simulink model "wamjc7"  (Simulink 8.3)
settings: Solver=ode4  SolverMode=SingleTasking  StartTime=0.0  StopTime=inf  FixedStep=sample_time  RelTol=1e-3
undefined symbols (not defined in the file): arm_home, arm_home_norest, arm_j2mt, arm_m2jp, b, bit, C, CAN_init, enc_per_rev, FT_init, hand_on, MT_init, puck_I_per_Nm, rotFT2Hand, sample_time, Standard, VL1_init, VL2_init
libraries: xpclib x43, simulink x27, xpcutilitieslib x6, dspmathops x1, dspadpt3 x1, dspindex x1, dspbuff3 x1
(part 4 of 5)

== matlab function Get Arm State/Get Gripper Status/Grasp Success ==
  data: isGraspMessage input double; grasp_success output double; errorcode input double
function grasp_success = f(isGraspMessage, errorcode)
%#eml

    persistent errorcode_last;
    
    if isempty(errorcode_last)
       errorcode_last = -1; 
    end

    grasp_success = 0;
    
    % If this is a grasp message, the current errorcode is a grasp succces 
    % and the previous one was not then return a success
    if isGraspMessage && errorcode == 0 && errorcode_last ~= 0
       grasp_success = 1; 
       errorcode_last = double(errorcode);
    elseif ~isGraspMessage
        errorcode_last = -1;
    end
    

end

== matlab function Subsystem/Plan Arm Trajectory/Determine parameters ==
  data: dt input double; x0 output double; xf output double; acc output double; vel output double; Tdes output double; pos output double; hand_on input double; x0_in input double; pckt input double; type output double; guarded output double; FT input double
% if joint space move, computes the trajectory using a trapezoidal velocity profile
% if cartesian space move, computes the trajectory using one selected position axis, and theta

% if joint space:
% x0,xf are start and end position in radians
%     type==0
% if cartesian space:
% x0,xf are start and end position in meters/radians
%     type==any other
function [x0,xf,acc,vel,Tdes,pos,type, guarded] = det_params(dt,hand_on,x0_in,pckt,FT)

    % This is used for compliant closing
    persistent initialGripperWidth;
    
    if(isempty(initialGripperWidth))
        initialGripperWidth = 0;
    end
    
    % parse the UDP packet
    % pckt(1) is a double but is converted to uint8 (mask1 mask2 mask3 mask4 mask5 type(3 bits))
    data = uint8(pckt(1));
    bits = bitand(bitshift(data,-7:0),1)';
    posMask = 2*bits(4)+bits(5);
    
    type = double(4*bits(6)+2*bits(7)+bits(8));
    guarded = [0 0 dt 0 0];
    % determine x0 (depends on cartesian space or joint space)
    % joint space move
    if(type == 0)
        acc = pckt(9:15);
        vel = pckt(16:22);
        xf  = pckt(2:8);
        
        Tdes = nan(4,4);
        x0 = x0_in;
        pos = nan(3,1);
        guarded = [0 0 dt 0 0];
    % cartesian space move
    elseif(type == 1)
        % acc and vel are unused for Jacobian Transpose controller
        acc = [.05 .05 .05 .05 0 0 0]';
        vel = [.1  .1  .1  .1  0 0 0]';
        % Unpack the transfomation matrix
        TF = [pckt(2)  pckt(3)  pckt(4)  pckt(5);
              pckt(6)  pckt(7)  pckt(8)  pckt(9);
              pckt(10) pckt(11) pckt(12) pckt(13);
              0 0 0 1;];
        Tdes = TF; % Entire transformation matrix describing desired tool configuration
        
        % Build the guarded signal from the packet
        guarded = [pckt(18) pckt(19) dt pckt(20) pckt(21)];
        
        pos = TF(1:3,4);  % Position part of transformation matrix describing the desired tool configuration
        
        % we need to compute the forward kinematics
        % to determine the initial tool configuration vector
        
        % a, d, and alpha (b) DH parameters
        dh_a = [0 0 0.045 -0.045 0 0 0 0];
        dh_d = [0 0 0.55 0 0.3 0 .061 0]; % Not sure about dh_d(8) For the hand
        dh_b = [-pi/2 pi/2 -pi/2 pi/2 -pi/2 pi/2 0 0];

        % hand on
        if (hand_on)
            dh_d(8) = 0.0953; % Schunk Gripper
        end

        % compute forward kinematics of initial position
        ct = cos([x0_in; 0]);
        st = sin([x0_in; 0]);
        cb = cos(dh_b);
        sb = sin(dh_b);        
        T0 = eye(4);
        for i=1:8
            T = [ ct(i), -st(i)*cb(i),  st(i)*sb(i), dh_a(i)*ct(i);
                  st(i),  ct(i)*cb(i), -ct(i)*sb(i), dh_a(i)*st(i);
                  0, sb(i), cb(i), dh_d(i);
                  0, 0, 0, 1 ];
            T0 = T0*T;
        end
        
        x0 = [T0(1:3,4)' 0 0 0 0]';
        xf = [pos' 0 0 0 0]';

    % A Trajectory Move
    elseif(type == 2)
        % Execute a trajectory given in the UDP packet.  There will be 100 points along the trajectory,
        % each with seven values (joints 1-7).  In the packet the points will start at pckt(PTS_START)
        
        acc = zeros(7,1);
        vel = zeros(7,1);
        pos = zeros(3,1);
        x0 = zeros(7,1);
        xf = zeros(7,1);
        
        PTS_START = 3;  

        % Get the length (in seconds) that the trajectory should take
        trajectoryEndTime = pckt(2);
        
        % Index of 100 points in the trajectory that the current time falls at
        index = (dt / trajectoryEndTime)*100;
        % The first point that we will want to interpolate between
        lowIndex = floor(index);
        % The distance between the two points (used for linear interpolation)
        alpha = index - lowIndex;
        
        % Get the start and end joint angles from the packet
        startIndex = lowIndex*7 + PTS_START;
        qStart = zeros(1,7);
        qEnd = zeros(1,7);
        qStart(1) = pckt(startIndex    );
        qStart(2) = pckt(startIndex + 1);
        qStart(3) = pckt(startIndex + 2);
        qStart(4) = pckt(startIndex + 3);
        qStart(5) = pckt(startIndex + 4);
        qStart(6) = pckt(startIndex + 5);
        qStart(7) = pckt(startIndex + 6);
        qEnd(1)   = pckt(startIndex + 7);
        qEnd(2)   = pckt(startIndex + 8);
        qEnd(3)   = pckt(startIndex + 9);
        qEnd(4)   = pckt(startIndex + 10);
        qEnd(5)   = pckt(startIndex + 11);
        qEnd(6)   = pckt(startIndex + 12);
        qEnd(7)   = pckt(startIndex + 13);

        % For some reason Matlab did not like the syntax:
        %  qStart = pckt(startIndex : startIndex + 6);
        %  qEnd   = pckt(startIndex + 7 : startIndex + 13);
        % or even
        %  qStart(1:7) = pckt(startIndex : startIndex + 6);
        
        % Do a linear interpolation between the two joint angles
        qdes = (1-alpha)*qStart + alpha*qEnd;
        
        %Pack the position into Tdes so we do not have to create another signal
        Tdes = zeros(4,4);
        Tdes(1:7) = qdes';
        
        % Put finised time in x0(1)
        x0(1) = trajectoryEndTime;
        
    % Compliant close.
    elseif type == 3       
        x0 = zeros(7,1);
        xf = zeros(7,1);
        acc = zeros(7,1);
        vel = zeros(7,1);
        pos = zeros(3,1);
        
        % If we are just at the beginning of a compliant close, get the
        % current gripper width as the starting gripper width
        if dt < .004
           %initialGripperWidth = FT(8); 
           initialGripperWidth = .1;
        end
        
        targetGripperWidth = pckt(2);
        gripperSpeed = pckt(3);
        finger = pckt(4);
        
        totalTime = abs(initialGripperWidth - targetGripperWidth) / gripperSpeed;
        
        % Get the fingertip position
        fingerTipPosition = finger*initialGripperWidth/2;
                
        % a, d, and alpha (b) DH parameters
        dh_a = [0 0 0.045 -0.045 0 0 0 0];
        dh_d = [0 0 0.55 0 0.3 0 .061 0]; % Not sure about dh_d(8) For the hand
        dh_b = [-pi/2 pi/2 -pi/2 pi/2 -pi/2 pi/2 0 0];

        % hand on
        if (hand_on)
            dh_d(8) = 0.0953; % Schunk Gripper
        end

        % compute forward kinematics of initial position
        ct = cos([x0_in; 0]);
        st = sin([x0_in; 0]);
        cb = cos(dh_b);
        sb = sin(dh_b);
        T0 = eye(4);
        for i=1:8
            T = [ ct(i), -st(i)*cb(i),  st(i)*sb(i), dh_a(i)*ct(i);
                  st(i),  ct(i)*cb(i), -ct(i)*sb(i), dh_a(i)*st(i);
                  0, sb(i), cb(i), dh_d(i);
                  0, 0, 0, 1 ];
            T0 = T0*T;
        end
        
        % Add the rotated vector from palm to fingertip
        T0(1:3,4) = T0(1:3,4) + T0(1:3,1:3)*[0;fingerTipPosition;.073];
        
        Tdes = T0;
        
        % Build the guarded signal
        guarded = [0 0 dt 0 0];
        
        % Get the time that the gripper should take to close
        x0(1) = totalTime;
        
        % The grasp success flag
        x0(2) = FT(9);
        
        % pos(1) pass which finger should remain stationary through to the
        % compute qdes,qddes block
        pos(1) = finger;
        
        % pos(2) holds the predicted gripper position
        pos(2) = initialGripperWidth - (dt/totalTime)*(initialGripperWidth - targetGripperWidth);
    elseif type == 5
        x0 = x0_in;
        xf = x0_in;
        acc = zeros(7,1);
        vel = zeros(7,1);
        Tdes = zeros(4,4);
        pos = zeros(3,1);
        guarded = [0 0 dt 0 0];
        vel(1) = pckt(2);  % Tf for an impedance move
    else
        x0 = x0_in;
        xf = x0_in;
        acc = zeros(7,1);
        vel = zeros(7,1);
        Tdes = zeros(4,4);
        pos = zeros(3,1);
        %type = 0;
    end
end

== matlab function Subsystem/Plan Arm Trajectory/Trapezoidal Profile2 ==
  data: dt input double; xdes output double; x0 input double; xf input double; acc input double; vel input double; xddes output double; done output double; type input double; cartesian_error input double; m output double
function [xdes,xddes,done,m] = trap_traj(dt,x0,xf,acc,vel,type,cartesian_error)
    % assume we're done
    done = 1;

    % initialize xdes and xddes
    xdes = zeros(7,1);
    xddes = zeros(7,1);
    m = [0.0 0.0 dt];

    if type == 0
        % iterate through joints
        for i=1:7
            % check if we're already done with this joint
            if(xf(i) == x0(i))
                xdes(i) = xf(i);
                % xddes(i) was initialized to 0
                continue;
            end

            % change acceleration and velocity to appropriate sign
            a = acc(i)*sign(xf(i)-x0(i));
            v = vel(i)*sign(xf(i)-x0(i));

            % t1,q1 are the time and position at the first peak of the trapezoid
            % t2,q2 are the time and position at the second peak of the trapezoid
            % v2 is the velocity at the midpoint of the trapezoid
            % qramp is the distance traveled during the acceleration phase
            % tmid is the time spent at constant velocity
            % tf is the total time to reach desired position (t1+t2+tmid)
            % a = vt; q = 0.5*a*t^2
            t1 = v/a;
            qramp = 0.5*a*t1^2;

            % acceleration is not high enough to reach our constant velocity, so trapezoid
            % looks like a triangle instead
            if (abs(2*qramp) > abs(xf(i)-x0(i)))
                % (xf-x0)/2 = 0.5*a*t^2
                t1 = sqrt((xf(i)-x0(i))/a);
                tmid = 0;
                qramp = (xf(i)-x0(i))/2;
                v2 = a*t1;
            % we will hit constant velocity, so trapezoid is really a trapezoid
            else
                tmid = (xf(i)-x0(i)-2*qramp)/v;
                v2 = v;
            end

            % compute the remaining params
            t2 = t1 + tmid;
            tf = t1*2 + tmid;
            q1 = x0(i) + qramp;
            q2 = q1 + v*tmid;

            % acceleration stage
            if (dt < t1)
                tloc = dt;
                xdes(i) = x0(i) + 0.5*a*tloc^2;
                xddes(i) = a*tloc;
            % constant velocity stage
            elseif (dt < t2)
                tloc = dt-t1;
                xdes(i) = q1 + v*tloc;
                xddes(i) = v;
            % deceleration stage
            elseif (dt < tf)
                tloc = dt-t2;
                xdes(i) = q2 + v2*tloc - 0.5*a*tloc*tloc;
                xddes(i) = -a*tloc+v2;
            % hold until next trajectory point
            else
                xdes(i) = xf(i);
                % xddes(i) was initialized to 0
            end

            % check if has finished yet
            if (dt < tf)
                done = 0;
            end
        end
    elseif type == 1  % Cartesian space move

        % This only determines if we have finished a cartesian space move.
        % A cartesian space move runs for at least .25 seconds and no more than 15 seconds.
        % If the time is witin these limits, a cartesian space move is done if the error is 
        % less than the bounds.
        
        % Run for at least .25 seconds
        if dt < .25
            done = 0;
        else
            m(1) = max(abs(cartesian_error(1:3)));
            m(2) = max(abs(cartesian_error(4:6)));
            % If we have been running for less than 15 seconds and we are still far away, we are not done.
            %if  dt < 15 && (norm(cartesian_error(1:3)) > .02 || norm(cartesian_error(4:6)) > .1)
            if  dt < 15 && ( m(1) > .01 || m(2) > .01)
                done = 0;
            else
                done = 1;
            end
        end
    % A trajectory move
    elseif type == 2
        if dt < x0(1)
            done = 0;
        end
        
    % A compliant close
    elseif type == 3
        
        % This only determines if we have finished a compliant close.
        % A compliant close runs for time specified for the gripper to close [in x0(1)].
        % If the current time is less than the maximum running time, a compliant close can 
        % be stopped if the gripper returns a grasp success, or if there is an error.
        
        % If we have been running for less than the time specified in x0(1)
        if  dt < x0(1)
            done = 0;
        else
            done = 1;
        end
        
        % If there was a grasp success
        if x0(2) == 1
            done = 1;
        end
        
    elseif type == 5
        
        % vel(1) has tf for an impedance move
        if dt > 1.1*vel(1)
            done = 1;
        else
            done = 0;
        end
       
    else
        done = 1;
    end
    
end

== matlab function Receive Controller Commands/Embedded MATLAB Function ==
  data: t input double; data input double; FTSIGNAL output double; TAUSIGNAL output double; rcvd input double
function [FTSIGNAL, TAUSIGNAL]  = fcn(t,data, rcvd)
%#eml
    
    persistent torque_percentage tausignal torque_state torque_duration torque_start_time taredTime biasStartTime
    % Values for torque_state
    %  0 : Torque is off (0%)
    %  1 : Torque is increasing
    % -1 : Torque is decreasing
    %  2 : Torque is full (100%)
    
    if isempty(torque_percentage) || isempty(tausignal) || isempty(torque_state) || isempty(torque_duration) || isempty(torque_start_time) || isempty(taredTime) || isempty(biasStartTime)
       torque_percentage = 0;
       tausignal = 0;
       torque_state = 0;
       torque_duration = 0;
       torque_start_time = 0;
       taredTime = 0;
       biasStartTime = -1;
    end

    tarenow = 0;
    biasFT = 0;
    readFT = 0;

    % If there is a new packet this cycle
    if(rcvd == 1)
        switch(data(1))  % Using a switch because we may want to implement other commands
            case 1 % Tare command
                tarenow = 1;
                taredTime = t;
            case 2 % Increase Torque Percentage to 100%
                % Can only increase the torque if it is off
                if torque_state == 0 && torque_percentage == 0
                    torque_state = 1;
                    torque_start_time = t;
                    torque_duration = double(data(2));
                end
            case 3 % Decrease Torque Percentage to 0%
                if torque_state == 2 && torque_percentage == 1
                    torque_state = -1;
                    torque_start_time = t;
                    torque_duration = double(data(2));
                end
            case 4 % Bias command
                biasStartTime = t;              

        end
    else
        if(t == .004) % Just starting the model
            tarenow = 1;
            taredTime = t;
        end
    end
    
    % Must calculate bias from .5 seconds to 1.5 seconds after sending the tare command
    % More than 1.5 seconds, do not calculate bias
    if(t - taredTime > 1.5)
        readFT = 1;
    end
    
    if(biasStartTime > 0 && t - biasStartTime <= 1)
        biasFT = 1;
    end

    % Put together the FTSIGNAL
    FTSIGNAL = [tarenow biasFT readFT];
    
    
    % Put together the TAUSIGNAL
    if torque_state == 1 % Increasing the torque
       dt = t - torque_start_time;
       if dt < torque_duration
          torque_percentage = dt/torque_duration;
       else
          torque_state = 2; % Reached full torque
          torque_percentage = 1;
       end
       
    elseif torque_state == -1 % Decreasing the torque
       dt = t - torque_start_time;
       if dt < torque_duration
          torque_percentage = 1 - dt/torque_duration;
       else
          torque_state = 0;
          torque_percentage = 0;
       end
    end
    
    TAUSIGNAL = torque_percentage;
end

== matlab function Subsystem/Plan Arm Trajectory/Send Execution Result/Determine Execution Result ==
  data: Done input double; DoneChanged input double; sendPacket output double; ExecutionStatus input double; result output double; contact input double; t input double
function [sendPacket, result] = getResult(Done, DoneChanged, ExecutionStatus, contact,t)
%#eml

    sendPacket = 0;
    startOrFinish = 0;
    executionResult = 0;
    result = [0 0 0 0 0 t];
    % result(1) - 1: Move started
    % result(1) - 2: Move finished
    
    % result(2) - only valid if result(1) == 2
    %             0 - Failure
    %             1 - Success
    %             2 - Need to start a compliant close
    
    result(3) = ExecutionStatus(1); % FTError
    result(4) = ExecutionStatus(2); % contact_or_not
    result(5) = ExecutionStatus(3); % contact_scenario

    if DoneChanged && ~Done    % We just started a move
       startOrFinish = 1; 
       sendPacket = 1;

    elseif contact(1) == 1
       startOrFinish = 2;
       sendPacket = 1;
       executionResult = 0;
       result(4) = contact(1);
       result(5) = contact(2);
       
    elseif (DoneChanged && Done) || ExecutionStatus(1) % We just finished a move
       startOrFinish = 2;
       sendPacket = 1;
       if ExecutionStatus(1)
           executionResult = 0;
       else
           executionResult = 1;
       end
       
    elseif contact(1) == 2  % If axis is blocked
        startOrFinish = 2;
        sendPacket = 1;
        executionResult = 2;
        result(3) = 0; % FTError;
        result(4) = 1; % contact_or_not
        % Turn left fingertip into left finger, and right fingertip into right finger
        if contact(2) == 1 % Left fingertip
          result(5) = 8; % Left finger
        elseif contact(2) == 2 % Right fingertip
          result(5) = 7; % Right finger
        elseif contact(2) == 4 % Palm
          result(5) = 4;
        end
    end

    result(1) = startOrFinish;
    result(2) = executionResult;
 
end

== matlab function Subsystem/MATLAB Function ==
  data: isNotImpOld input double; pckt input double; q input double; isNotImp output double; ImpData output double; time input double; t_s output double; xi output double; qi output double
function [isNotImp, ImpData,t_s,xi,qi] = fcn(isNotImpOld,pckt,q,time)
%#codegen
    data = uint8(pckt(1));
    bits = bitand(bitshift(data,-7:0),1)';
    
    type = double(4*bits(6)+2*bits(7)+bits(8));
    
    persistent t_start pos_i quat_i;
    if isempty(t_start) || isempty(quat_i) || isempty(pos_i);
        t_start = 0;
        pos_i = [0 0 0]';
        quat_i = [1 0 0 0]';
    end
    
    
    if(type==5)
        isNotImp = 0;
        ImpData = pckt(2:30)';
    else
        isNotImp =1;
        ImpData = zeros(1,29);
    end
    
    if xor(isNotImpOld,isNotImp)
        t_start = time;
        tf = fkWam7(q);
        pos_i = tf(1:3,4);
        quat_i = r2quat(tf);
        
    end
   t_s = t_start;
   qi = quat_i;
   xi = pos_i;

end

function A07 = fkWam7(q)
% Put origin of Frame 7 at intersection of wrist axes.
%syms a3 d3 d5 
a3 = 0.045;  d3 = 0.55;  d5 = 0.3;   d7 = 0.1563;
A01 = trotz(q(1))                   * round(trotx(-pi/2));
A12 = trotz(q(2))                   * round(trotx(pi/2)) ;
A23 = trotz(q(3)) * transl(a3,0,d3) * round(trotx(-pi/2));
A34 = trotz(q(4)) * transl(-a3,0,0) * round(trotx(pi/2)) ;
A45 = trotz(q(5)) * transl(0,0,d5)  * round(trotx(-pi/2));
A56 = trotz(q(6))                   * round(trotx(pi/2)) ;
A67 = trotz(q(7)) *transl(0,0,d7)                        ;
A07 = A01 * A12 * A23 * A34 * A45 * A56 * A67;

end
function [unit_quat] = r2quat(t)
    qs = sqrt(trace(t))/2.0;
    kx = t(3,2) - t(2,3);   % Oz - Ay
    ky = t(1,3) - t(3,1);   % Ax - Nz
    kz = t(2,1) - t(1,2);   % Ny - Ox

    if (t(1,1) >= t(2,2)) & (t(1,1) >= t(3,3)) 
        kx1 = t(1,1) - t(2,2) - t(3,3) + 1; % Nx - Oy - Az + 1
        ky1 = t(2,1) + t(1,2);          % Ny + Ox
        kz1 = t(3,1) + t(1,3);          % Nz + Ax
        add = (kx >= 0);
    elseif (t(2,2) >= t(3,3))
        kx1 = t(2,1) + t(1,2);          % Ny + Ox
        ky1 = t(2,2) - t(1,1) - t(3,3) + 1; % Oy - Nx - Az + 1
        kz1 = t(3,2) + t(2,3);          % Oz + Ay
        add = (ky >= 0);
    else
        kx1 = t(3,1) + t(1,3);          % Nz + Ax
        ky1 = t(3,2) + t(2,3);          % Oz + Ay
        kz1 = t(3,3) - t(1,1) - t(2,2) + 1; % Az - Nx - Oy + 1
        add = (kz >= 0);
    end

    if add
        kx = kx + kx1;
        ky = ky + ky1;
        kz = kz + kz1;
    else
        kx = kx - kx1;
        ky = ky - ky1;
        kz = kz - kz1;
    end
    nm = norm([kx ky kz]);
    if nm == 0
        unit_quat = [1 0 0 0]';
    else
        s = sqrt(1 - qs^2) / nm;
        qv = s*[kx ky kz];
        
        unit_quat = [qs qv]';

    end
end

== matlab function Subsystem/Impedance Controller/Split up parameters ==
  data: quatf output double; xf output double; axis output double; theta output double; data input double; tf output double; qi input double; poff output double; Const output double; Fp output double; R output double
function [quatf,xf,axis,theta,tf,poff,Const,Fp,R] = getParams(data,qi)
%#codegen
tf = data(1)';
xf = data(2:4)';
quatf = data(5:8)';
poff = data(9:11)';
Const = data(12:17)';
Fp = data(18:20)';
quat = quatprod(qi,qinv(quatf));
theta = 2*atan2(norm(quat(2:4)),quat(1));
axis = quat(1:3) ./sin(theta/2);

R = zeros(3,3);
R(1,1) = data(21);
R(1,2) = data(22);
R(1,3) = data(23);
R(2,1) = data(24);
R(2,2) = data(25);
R(2,3) = data(26);
R(3,1) = data(27);
R(3,2) = data(28);
R(3,3) = data(29);

if(theta>pi)
    theta = 2*pi - theta;
    quatf=qinv(quatf);
elseif(theta<-pi)
    theta = 2*pi + theta;
    quatf=qinv(quatf);
end



end

function qi = qinv(q)

qi = [q(1);-q(2);-q(3);-q(4)];
end
function product = quatprod(q1,q2)
product = [q1(1)*q2(1)-q1(2:4)'*q2(2:4); q1(1)*q2(2:4)+q2(1)*q1(2:4)+cross(q1(2:4),q2(2:4))];

end

== matlab function Subsystem/Impedance Controller/Impedance Torque Caclutation ==
  data: x0 input double; tauapp output double; v0 input double; a0 input double; q input double; qd input double; K input double; B input double; Md input double; M input double; nonLinear input double; poff input double; deltax output double; Cons input double; Fe output double; Fp input double; R input double
function [tauapp,deltax,Fe]= impedanceControl(x0, v0, a0,q, qd,K,B,Md ,M,nonLinear,poff,Cons,Fp,R)
%Impedance Controller
%x0,v0,a0 are the desired position, velocity, acceleration
%q qd are joint positions and velocities
%K is stiffness matrix
%B is damping matrix
%Md is the controller inertia matrix
%M is the inertia mass matrix in the lagrange equation M(q)
%nonLinear is sum of C(q,qd) and G(q) terms

%Find Jacobians and positional error
tf = fkWam7(q,poff);
[J,~]=Jdot(q,zeros(7,1),poff);
Jd = jacob_dot(q,qd,poff);
x = [tf(1:3,4);r2quat(tf)];
xquat = [sqrt(1-norm(x0(4:6))^2);x0(4:6)];
dx = quatprod(xquat,qinv(r2quat(tf)));
if(dx(1)<0)
    dx = -dx;
end

deltax = [x0(1:3)-x(1:3);dx(2:4)];

rotmat = [R' zeros(3,3); zeros(3,3) R'];
K = diag([Cons(1) Cons(2) Cons(3) Cons(4) Cons(5) Cons(6)])*rotmat;
%K = K*blkdiag(R,eye(3));
B = diag([1 1 1 1 1 1])*rotmat;
Md= diag([4 4 4 4 4 4])*rotmat;

K(4:6,4:6) = 2*(dx(1)*eye(3)+S(dx(2:4)))*K(4:6,4:6);
Fa = [Fp ; 0 ; 0 ; 0];

%internal motion damping
kd = .1;
[val,ind] = max(qd);
ns = null(J);
ns = ns(:,1);
taud = -kd*ns*val*sign(ns(ind));


%Impedance Control Law
Fe = eye(6)/Md*(Md*a0-Md*Jd(:,1)+B*(v0-J*qd)+K*(deltax))+Fa;
%Fe = B*(v0-J*qd)+K*(deltax);

%Calculate Torque
PinvJ= J';%/(J*J');
%taue = M*PinvJ*Fe;
taue = PinvJ*Fe;
%taue = taue - taue'*ns/norm(ns)^2;
%taue = M*J'*Fe;

%Add C(q,qd) and G(q) terms
tauapp= taue + nonLinear;%+frictionComp(qd);% +taud; 


Fe = [x0(4:6) ;deltax(4:6)];%%%%%%%%%%%%%%%%%%%%%%%%%%%%%%%%%%%%%%%%%%%%%%%%%%%%%%%%%*************************************************%%%%%%%%%%%%%%%%%%%%%

    
    
    
    
end


function A07 = fkWam7(q,poff)
% Put origin of Frame 7 at intersection of wrist axes.
%syms a3 d3 d5 
a3 = 0.045;  d3 = 0.55;  d5 = 0.3;   d7 = 0.1563;
A01 = trotz(q(1))                   * round(trotx(-pi/2));
A12 = trotz(q(2))                   * round(trotx(pi/2)) ;
A23 = trotz(q(3)) * transl(a3,0,d3) * round(trotx(-pi/2));
A34 = trotz(q(4)) * transl(-a3,0,0) * round(trotx(pi/2)) ;
A45 = trotz(q(5)) * transl(0,0,d5)  * round(trotx(-pi/2));
A56 = trotz(q(6))                   * round(trotx(pi/2)) ;
A67 = trotz(q(7)) * transl(poff(1),poff(2),poff(3)+d7)   ;
A07 = A01 * A12 * A23 * A34 * A45 * A56 * A67;

end

%%%%Edited Peter Corke's%%%%%%%%%%%%%%%%%%%%%%%%%%%%%%%%%%%%%%%%%%%%%%%%%%%
function [J,Jd] = Jdot(q,qd,poff)


	n = 7;
	
    Tj = eye(4);     % this is cumulative transform from base
    w = [0;0;0];
    v = [0;0;0];
    vel = zeros(3,n);
    omega = vel;
    R = zeros(3,3,n);
    T = R;
    p = vel;
    z = vel;
    J = zeros(6,n);
    Jd = J;
    
    a3 = 0.045;  d3 = 0.55;  d5 = 0.3;   d7 = 0.1563;
    
    for j=1:n,
        Aj=eye(4);
        switch j
            case 1
                Aj =  trotz(q(1))                   * round(trotx(-pi/2));
            case 2
                Aj = trotz(q(2))                   * round(trotx(pi/2)) ;
            case 3
                Aj = trotz(q(3)) * transl(a3,0,d3) * round(trotx(-pi/2));
            case 4
                Aj = trotz(q(4)) * transl(-a3,0,0) * round(trotx(pi/2)) ;
            case 5
                Aj = trotz(q(5)) * transl(0,0,d5)  * round(trotx(-pi/2));
            case 6
                Aj = trotz(q(6))                   * round(trotx(pi/2)) ;
            case 7
                Aj = trotz(q(7)) *transl(poff(1),poff(2),poff(3)+d7)                        ;
        end
        
        Tj = Tj * Aj;
        R(:,:,j) = Aj(1:3,1:3);
        T(:,:,j) = Tj(1:3,1:3);
        p(:,j) = Tj(1:3,4);    % origin of link j

        if j>1,
            z(:,j) = T(:,:,j-1) * [0 0 1]'; % in world frame
            w = R(:,:,j)*( w + z(:,j) * qd(j));
            v = v + cross(R(:,:,j)*w, R(:,:,j-1)*p(:,j));
            %v = R{j-1}'*v + cross(w, p(:,j));
            %w = R{j-1}'* w + z(:,j) * qd(j);
        else
            z(:,j) = [0 0 1]';
            v = [0 0 0]';
            w = z(:,j) * qd(j);
        end

        vel(:,j) = v;       % velocity of origin of link j

        omega(:,j) = w;         % omega of link j in link j frame
    end
    

    
    for j=1:n,
        if j>1,
            t = p(:,n) - p(:,j-1);
            td = vel(:,n) - vel(:,j-1);
        else
            t = p(:,n);
            td = vel(:,n);
        end
       
            J_col = [cross(z(:,j), t); z(:,j)];
            Jdot_col = [cross(cross(omega(:,j), z(:,j)), t) + cross(z(:,j), td) ; cross(omega(:,j),  z(:,j))];
       

        J(:,j) = J_col;
        Jd(:,j) = Jdot_col;

    end
    A = Tj(1:3,1:3);
    %Je = [A,zeros(3);zeros(3),A]*J;
    w = J*qd;  %------change here
    Ad  = S(w(4:6))*A;
    Jd = [Ad,zeros(3);zeros(3),Ad]*J+[A,zeros(3);zeros(3),A]*Jd;
    8;
end

function [unit_quat] = r2quat(t)
    qs = sqrt(trace(t))/2.0;
    kx = t(3,2) - t(2,3);   % Oz - Ay
    ky = t(1,3) - t(3,1);   % Ax - Nz
    kz = t(2,1) - t(1,2);   % Ny - Ox

    if (t(1,1) >= t(2,2)) & (t(1,1) >= t(3,3)) 
        kx1 = t(1,1) - t(2,2) - t(3,3) + 1; % Nx - Oy - Az + 1
        ky1 = t(2,1) + t(1,2);          % Ny + Ox
        kz1 = t(3,1) + t(1,3);          % Nz + Ax
        add = (kx >= 0);
    elseif (t(2,2) >= t(3,3))
        kx1 = t(2,1) + t(1,2);          % Ny + Ox
        ky1 = t(2,2) - t(1,1) - t(3,3) + 1; % Oy - Nx - Az + 1
        kz1 = t(3,2) + t(2,3);          % Oz + Ay
        add = (ky >= 0);
    else
        kx1 = t(3,1) + t(1,3);          % Nz + Ax
        ky1 = t(3,2) + t(2,3);          % Oz + Ay
        kz1 = t(3,3) - t(1,1) - t(2,2) + 1; % Az - Nx - Oy + 1
        add = (kz >= 0);
    end

    if add
        kx = kx + kx1;
        ky = ky + ky1;
        kz = kz + kz1;
    else
        kx = kx - kx1;
        ky = ky - ky1;
        kz = kz - kz1;
    end
    nm = norm([kx ky kz]);
    if nm < 1e-3
        unit_quat = [1 0 0 0]';
    else
        s = sqrt(1 - qs^2) / nm;
        qv = s*[kx ky kz];
        
        unit_quat = [qs qv]';

    end
end

function qi = qinv(q)

qi = [q(1);-q(2);-q(3);-q(4)];
end
function product = quatprod(q1,q2)
product = [q1(1)*q2(1)-q1(2:4)'*q2(2:4); q1(1)*q2(2:4)+q2(1)*q1(2:4)+cross(q1(2:4),q2(2:4))];

end

function cros = S(v)
v1 = v(1);v2 = v(2);v3 = v(3);
cros = [0 -v3 v2;v3 0 -v1;-v2 v1 0];
end

function Jdot = jacob_dot( q, qd,poff)

	n = 7;
    
    % Using the notation of Angeles:
    %   [Q,a] ~ [R,t] the per link transformation
    %   P ~ R   the cumulative rotation t2r(Tj) in world frame
    %   e       the last column of P, the local frame z axis in world coordinates
    %   w       angular velocity in base frame
    %   ed      deriv of e
    %   r       is distance from final frame
    %   rd      deriv of r
    %   ud      ??
    
    % ^ aweful documentation 
    Q = zeros(3,3,7);
    P = zeros(3,3,7);
    a = zeros(3,7);
    e = zeros(3,7);
    w = zeros(3,7);
    ed = zeros(3,7);
    rd = zeros(3,7);
    r = zeros(3,7);
    ud = zeros(3,7);
    v = zeros(6,7);
    
    a3 = 0.045;  d3 = 0.55;  d5 = 0.3;   d7 = 0.1563;

    for i=1:n
        T = eye(4);
        switch i
            case 1
                T =  trotz(q(1))                   * round(trotx(-pi/2));
            case 2
                T = trotz(q(2))                   * round(trotx(pi/2)) ;
            case 3
                T = trotz(q(3)) * transl(a3,0,d3) * round(trotx(-pi/2));
            case 4
                T = trotz(q(4)) * transl(-a3,0,0) * round(trotx(pi/2)) ;
            case 5
                T = trotz(q(5)) * transl(0,0,d5)  * round(trotx(-pi/2));
            case 6
                T = trotz(q(6))                   * round(trotx(pi/2)) ;
            case 7
                T = trotz(q(7)) *transl(poff(1),poff(2),poff(3)+d7)    ;
        end
        Q(:,:,i) = T(1:3,1:3);
        a(:,i) = T(1:3,4);
    end

    P(:,:,1) = Q(:,:,1);
    e(:,i) = [0 0 1]';
    for i=2:n
        P(:,:,i) = P(:,:,i-1)*Q(:,:,i);
        e(:,i) = P(:,3,i);
    end

    % step 1
    w(:,1) = qd(1)*e(:,1);
    for i=1:(n-1)
        w(:,i+1) = qd(i+1)*[0 0 1]' + Q(:,:,i)'*w(:,i);
    end

    % step 2
    ed(:,1) = [0 0 0]';
    for i=2:n
        ed(:,i) = cross(w(:,i), e(:,i));
    end

    % step 3
    rd(:,n) = cross( w(:,n), a(:,n));
    for i=(n-1):-1:1
        rd(:,i) = cross(w(:,i), a(:,i)) + Q(:,:,i)*rd(:,i+1);
    end

    r(:,n) = a(:,n);
    for i=(n-1):-1:1
        r(:,i) = a(:,i) + Q(:,:,i)*r(:,i+1);
    end

    ud(:,1) = cross(e(:,1), rd(:,1));
    for i=2:n
        ud(:,i) = cross(ed(:,i), r(:,i)) + cross(e(:,i), rd(:,i));
    end

    % step 4
    %  swap ud and ed
    v(:,n) = qd(n)*[ud(:,n); ed(:,n)]; %me: look at size of this one
    for i=(n-1):-1:1
        Ui = [Q(:,:,i),zeros(3);zeros(3), Q(:,:,i)];
        v(:,i) = qd(i)*[ud(:,i); ed(:,i)] + Ui*v(:,i+1);
    end

    Jdot = v(:,1);
end
function bq = frictionComp(qd)
%parameters and model from paper http://homepages.inf.ed.ac.uk/svijayak/publications/mitrovic-ICRA2010.pdf
%Optimal Feedback Control for Anthropomorphic Manipulators
%Djordje Mitrovic, Sho Nagashima, Stefan Klanke, Takamitsu Matsubara, Sethu Vijayakumar
%ICRA 2010


s=20;
bc = [2.516 2.581 2.038 0.956 0.323 0.315 0.066]';
B =  [1.142 0.946 0.309 0.255 0.025 0.039 0.004]';

bq = bc.*atan(s*qd)*2/pi+B.*qd;
end

== matlab function Subsystem/Impedance Controller/Impedance Trajectory Generator ==
  data: quat0 input double; quat1 input double; xi input double; xf input double; axis input double; theta input double; tf input double; b input double; poff input double; t input double; xdes output double; vdes output double; ades output double; t_start input double; done output double
function [xdes,vdes,ades,done] = makeTraj(quat0,quat1,xi,xf,axis, theta,tf,b,poff,t,t_start)
%quat0 and quat1 are initial and final quaternions
%xi and xf are inital and final position vectors
%axis is the axis along any rotaion occurs
%theta is the rotation around the axis in radians
%b is the coefficients of the polynomial spline
%tf is the time that the spline takes
%t is time

t = t - t_start;



if t<tf
    %Calculate spline parameter F = [0,1] as t = [0,tf]
    F =   [t^5 t^4 t^3 t^2 t ]*b;
    Fd =  [5*t^4 4*t^3 3*t^2 2*t 1]*b;
    Fdd = [20*t^3 12*t^2 6*t 2 0]*b;
    


    %Calculate orientational quaternion
    omega = theta/2;
    
    if omega>1e-3
    xr = (sin((1-F)*omega)*quat0 +sin(F*omega)*quat1)/sin(omega);
    else
        xr = quat0;
        axis = [1;0;0];
    end
    xr=xr/norm(xr);
    %Calculate desired angular velocity and acceleration
    vr = -Fd*axis*theta;
    ar = -Fd*axis*theta;

    %Calculate position and 1st and 2nd derivatives
    xp = xi+F*(xf-xi)+quatRot(xr)*poff;
    vp = Fd*(xf-xi);
    ap = Fdd*(xf-xi);
    
    %Put parts together
    xdes= [xp;xr(2:4)];
    vdes= [vp;vr];
    ades= [ap;ar];
else
    %End of trajectory static condition
    xdes= [xf+quatRot(quat1)*poff;quat1(2:4)];
    vdes= [0;0;0;0;0;0];
    ades= [0;0;0;0;0;0];
end
if t>1.1*tf
    done = 1;
else 
    done = 0;
end

end


function [R] = quatRot(unit_q)
e0=unit_q(1);e1=unit_q(2);e2=unit_q(3);e3=unit_q(4);
R= [1-2*(e2^2+e3^2),2*(e1*e2-e3*e0),2*(e1*e3+e2*e0);
    2*(e1*e2+e3*e0),1-2*(e1^2+e3^2),2*(e2*e3-e1*e0);
    2*(e1*e3-e2*e0),2*(e2*e3+e0*e1),1-2*(e2^2+e1^2)];
end

== matlab function Subsystem/Impedance Controller/Polynomial Spline Generator ==
  data: coeff output double; tf input double
function coeff   = SplinePoly( tf)
%Assume inital and final velocities and accelerations equal to 0
v0=0;a0=0;vf=0;af=0;

%Ax = b where x is the coeffients of a 5th order polynonial where p(0)=0
A = [0 0 0 0 1; 0 0 0 2 0; tf^5 tf^4 tf^3 tf^2 tf ; 5*tf^4 4*tf^3 3*tf^2 2*tf 1 ; 20*tf^3 12*tf^2 6*tf 2 0];
b = [v0 ;a0; 1; vf; af];

%Solve for coefficients 
%If A is non square or singular use A'*A\(A'*b);
coeff = A\b;


%Maximum values of velocity and acceleration
%vmax = [5*(tf/2)^4 4*(tf/2)^3 3*(tf/2)^2 2*(tf/2) 1]*coeff;
%amax = [20*(tf/4)^3 12*(tf/4)^2 6*(tf/4) 2 0] * coeff;
end

== matlab function Subsystem/Plan Arm Trajectory/Verify ==
  data: qdes output double; qddes output double; qdes_in input double; qddes_in input double; error output double
function [qdes,qddes,error] = verify_q(qdes_in, qddes_in)

    % Assume no error
    error = 0;
    qdes = qdes_in;
    qddes = qddes_in;

%     % Check joint limits
    %qlim = [-2.62, 2.62; -2.01, 2.01; -2.97, 2.97; -0.87, 3.14; -4.79, 1.27; -1.57, 1.57; -3.0, 3.0;]; % Normal limits
    qlim = [-2.62, 2.62; -2.01, 2.01; -2.97, 2.97; -0.87, 3.14; -4.79, 1.27; -1.57, 1.57; -2.2146, 3.7854;]; % Limits with Schunk gripper attached
    qdlim = [1.01 1.01 1.01 1.01 1.01 1.01 1.01];
%     %if sum( qdes_in < qlim(:,1) ) ~= 7 || sum( qdes_in > qlim(:,2) ) ~= 7
%     %    error = 1;
%     %end
    % Set all out of range joint angles to eps inside the boundary, raise an error
    eps1 = 0; % Distance from joint angle that is considered an error
    eps2 = .01; % Amount to set joint towards zero away from error boundary
    for i = 1:7
        % Check lower boundary
        if qdes_in(i) < qlim(i,1) + eps1;
           qdes(i) = qlim(i,1) + eps1 + eps2; 
           error = 1;
        % Check upper boundary
        elseif qdes_in(i) > qlim(i,2) - eps1;
           qdes(i) = qlim(i,2) - eps1 - eps2;
           error = 1;
        end
        
        % Check joint velocity.  If any one is out of range, set desired velocity for all joints to zero
        if abs(qddes_in(i)) > qdlim(i)
            qddes = zeros(7,1);
            error = 1;
        end
    end

end

== matlab function Subsystem/Impedance Controller/Dynamics Compensation ==
  data: hand_on input double; tau output double; q input double; qd input double; qdd input double; FTsensor output double
function [tau, FTsensor] = dynamicsComp(hand_on,q,qd,qdd)
%-------------------------------------------------------------------------------------
%   SETUP THE ARM
%-------------------------------------------------------------------------------------    
    DH_a = [0 0 0.045 -0.045 0 0 0];
    DH_d = [0 0 .55 0 0.3 0 0.061];
    DH_alpha = [-pi/2 pi/2 -pi/2 pi/2 -pi/2 pi/2 0];

    m = [8.3936 4.8487 1.7251 2.17266212 0.35655692 0.40915886 0.07548270];
    
    com = zeros(3,7);
    com(:,1) = [0.3506e-3, 132.6795e-3, 0.6286e-3];
    com(:,2) = [-0.2230e-3, -21.3924e-3, 13.3754e-3];
    com(:,3) = [-38.7565e-3, 217.9078e-3, 0.0252e-3];
    com(:,4) = [0.00553408,0.00006822,0.11927695];
    com(:,5) = [0.00005483,0.02886286,0.00148493];
    com(:,6) = [-0.00005923,-0.01686123,0.02419052];
    com(:,7) = [ 0.00014836,0.00007252,-0.00335185];
    
    % Need Inertia matricies
    I = zeros(3,3,7);
    I(:,:,1) = [ 95157.4294e-6,   246.1404e-6,   -95.0183e-6 ;
                   246.1404e-6, 92032.3524e-6,  -962.6725e-6 ;
                   -95.0183e-6,  -962.6725e-6, 59290.5997e-6 ];
    I(:,:,2) = [ 29326.8098e-6,   -43.3994e-6,  -129.2942e-6 ;
                   -43.3994e-6, 20781.5826e-6,  1348.6924e-6 ;
                  -129.2942e-6,  1348.6924e-6, 22807.3271e-6 ];
    I(:,:,3) = [ 56662.2970e-6, -2321.6892e-6,     8.2125e-6 ;
                 -2321.6892e-6,  3158.0509e-6,   -16.6307e-6 ;
                     8.2125e-6,   -16.6307e-6, 56806.6024e-6 ];
    I(:,:,4) = [  0.01067491,  0.00004503, -0.00135557 ;
                  0.00004503,  0.01058659, -0.00011002 ;
                 -0.00135557, -0.00011002,  0.00282036 ];
    I(:,:,5) = [  0.00037112, -0.00000008, -0.00000003 ;
                 -0.00000008,  0.00019434, -0.00001613 ;
                 -0.00000003, -0.00001613,  0.00038209 ];
    I(:,:,6) =  [  0.00054889,  0.00000019, -0.00000010 ;
                   0.00000019,  0.00023846, -0.00004430 ;
                  -0.00000010, -0.00004430,  0.00045133 ];
    I(:,:,7) = [ 0.00003911, 0.00000019, 0.00000000 ;      % WAM without hand
                 0.00000019, 0.00003877, 0.00000000 ;
                 0.00000000, 0.00000000, 0.00007614 ];
    
    %Link Gear Ratio
    % The differential drive mechanism was ignored here because it's not
    % supported by the robotic toolbox yet.
    % Please refer to: http://www.me.unm.edu/~starr/research/WAM_MassParams_AA-00.pdf
    G = zeros(7,1);
    G(1) =  42.00;
    G(2) =  28.25;
    G(3) =  28.25;
    G(4) =  18.00;
    G(5) =  9.70;
    G(6) =  9.70;
    G(7) =  14.93;
    %Link Motor Inertia
    Jm = zeros(7,1);
    Jm(1) = 0.00011631;
    Jm(2) = 0.00011831;
    Jm(3) = 0.00011831;
    Jm(4) = 0.00010686;
    Jm(5) = 0.00001685;
    Jm(6) = 0.00001745;
    Jm(7) = 0.00000142;
             
    if hand_on
        hand_mass = 1.385;
        DH_d(7) = DH_d(7) + .0953; % Adding the distance to the hand frame for the Schunk Gripper
        com(:,7) = ([0.001127;	-0.000211;	0.054851].*hand_mass + com(:,7).*m(7))/(hand_mass + m(7)); % Finding the combined center of mass
        m(7) = m(7) + hand_mass; % Adding the mass of the hand
        I(:,:,7) = [ .003167342,          0,         0;       % Approximate Inertia Tensor for Schunk Gripper
                              0, .001128942,         0;
                              0,          0, .00258007;];
    end
    
%-------------------------------------------------------------------------------------
%  END SETUP OF THE ARM
%-------------------------------------------------------------------------------------

    z0 = [0;0;1];
    grav = [0 0 9.81];
	fext = zeros(6, 1);
    n = 7;
    FTsensor = zeros(6,1);
    
    tau = zeros(n,1);
    
    Fm = zeros(3,7);
    Nm = zeros(3,7);
    N = zeros(3,1);
    pstarm = zeros(3,7);
    Rm = zeros(3,3,7);
    w = zeros(3,1);
    wd = zeros(3,1);
    v = zeros(3,1);
    vd = grav(:);
    
    
    %
	% init some variables, compute the link rotation matrices
	%
    for j=1:n,
        a = DH_a(j);
        d = DH_d(j);
        alpha = DH_alpha(j);
        Tj = getTransformDH(a, d, alpha, q(j));
        
        pstar = [a; d*sin(alpha); d*cos(alpha)];
        if j == 1,
            pstar = eye(3) * pstar;
            Tj = eye(4) * Tj;
        end
        pstarm(:,j) = pstar;
        Rm(:,:,j) = Tj(1:3,1:3);
    end
    
    %
	%  the forward recursion
	%
    for j=1:n,
        Rt = Rm(:,:,j)';	% transpose!!
        pstar = pstarm(:,j);
        r = com(:,j)';

        %
        % statement order is important here
        %
        % revolute axis
        wd = Rt*(wd + z0*qdd(j) + cross(w,z0*qd(j)));
        w = Rt*(w + z0*qd(j));
        %v = cross(w,pstar) + Rt*v;
        vd = cross(wd,pstar) + cross(w, cross(w,pstar)) + Rt*vd;

        %vhat = cross(wd,r') + cross(w,cross(w,r')) + vd;
        vhat = cross(wd,r') + cross(w,cross(w,r')) + vd;
        F = m(j)*vhat;
        N = I(1:3,1:3,j)*wd + cross(w,I(1:3,1:3,j)*w);
        Fm(:,j) = F;
        Nm(:,j) = N;
    end
    
    
    %
	%  the backward recursion
	%

    fext = fext(:);
    f = fext(1:3);		% force/moments on end of arm
    nn = fext(4:6);

    for j=n:-1:1,
        pstar = pstarm(:,j);

        %
        % order of these statements is important, since both
        % nn and f are functions of previous f.
        %
        if j == n,
            R = eye(3,3);
        else
            R = Rm(:,:,j+1);
        end
        r = com(:,j)';
        
        % The expected force/torque at the sensor.  Used for dynamic compensation
        % of the gripper.
        if j == n
            FTsensor(1:3) = R*f + Fm(:,j);
            FTsensor(4:6) = cross(r',Fm(:,j));
        end
        
        nn = R*(nn + cross(R'*pstar,f)) + cross(pstar+r',Fm(:,j)) + Nm(:,j);
        f = R*f + Fm(:,j);
        
        R = Rm(:,:,j);
        % revolute
        tau(j) = nn'*(R'*z0) + G(j)^2 * Jm(j)*qdd(j);% + abs(G(j)) * friction(link, qd(j));
    end

end

function T = getTransformDH(a,d,alpha,q)
    ct = cos(q);
    st = sin(q);
    cb = cos(alpha);
    sb = sin(alpha);
    
    T = [ ct, -st*cb,  st*sb, a*ct;
          st,  ct*cb, -ct*sb, a*st;
          0, sb, cb, d;
          0, 0, 0, 1 ];
end

== matlab function Subsystem/Impedance Controller/Subsystem1/Dynamics Compensation ==
  data: hand_on input double; tau output double; q input double; qd input double; qdd input double; FTsensor output double
function [tau, FTsensor] = dynamicsComp(hand_on,q,qd,qdd)
%-------------------------------------------------------------------------------------
%   SETUP THE ARM
%-------------------------------------------------------------------------------------    
    DH_a = [0 0 0.045 -0.045 0 0 0];
    DH_d = [0 0 .55 0 0.3 0 0.061];
    DH_alpha = [-pi/2 pi/2 -pi/2 pi/2 -pi/2 pi/2 0];

    m = [8.3936 4.8487 1.7251 2.17266212 0.35655692 0.40915886 0.07548270];
    
    com = zeros(3,7);
    com(:,1) = [0.3506e-3, 132.6795e-3, 0.6286e-3];
    com(:,2) = [-0.2230e-3, -21.3924e-3, 13.3754e-3];
    com(:,3) = [-38.7565e-3, 217.9078e-3, 0.0252e-3];
    com(:,4) = [0.00553408,0.00006822,0.11927695];
    com(:,5) = [0.00005483,0.02886286,0.00148493];
    com(:,6) = [-0.00005923,-0.01686123,0.02419052];
    com(:,7) = [ 0.00014836,0.00007252,-0.00335185];
    
    % Need Inertia matricies
    I = zeros(3,3,7);
    I(:,:,1) = [ 95157.4294e-6,   246.1404e-6,   -95.0183e-6 ;
                   246.1404e-6, 92032.3524e-6,  -962.6725e-6 ;
                   -95.0183e-6,  -962.6725e-6, 59290.5997e-6 ];
    I(:,:,2) = [ 29326.8098e-6,   -43.3994e-6,  -129.2942e-6 ;
                   -43.3994e-6, 20781.5826e-6,  1348.6924e-6 ;
                  -129.2942e-6,  1348.6924e-6, 22807.3271e-6 ];
    I(:,:,3) = [ 56662.2970e-6, -2321.6892e-6,     8.2125e-6 ;
                 -2321.6892e-6,  3158.0509e-6,   -16.6307e-6 ;
                     8.2125e-6,   -16.6307e-6, 56806.6024e-6 ];
    I(:,:,4) = [  0.01067491,  0.00004503, -0.00135557 ;
                  0.00004503,  0.01058659, -0.00011002 ;
                 -0.00135557, -0.00011002,  0.00282036 ];
    I(:,:,5) = [  0.00037112, -0.00000008, -0.00000003 ;
                 -0.00000008,  0.00019434, -0.00001613 ;
                 -0.00000003, -0.00001613,  0.00038209 ];
    I(:,:,6) =  [  0.00054889,  0.00000019, -0.00000010 ;
                   0.00000019,  0.00023846, -0.00004430 ;
                  -0.00000010, -0.00004430,  0.00045133 ];
    I(:,:,7) = [ 0.00003911, 0.00000019, 0.00000000 ;      % WAM without hand
                 0.00000019, 0.00003877, 0.00000000 ;
                 0.00000000, 0.00000000, 0.00007614 ];
    
    %Link Gear Ratio
    % The differential drive mechanism was ignored here because it's not
    % supported by the robotic toolbox yet.
    % Please refer to: http://www.me.unm.edu/~starr/research/WAM_MassParams_AA-00.pdf
    G = zeros(7,1);
    G(1) =  42.00;
    G(2) =  28.25;
    G(3) =  28.25;
    G(4) =  18.00;
    G(5) =  9.70;
    G(6) =  9.70;
    G(7) =  14.93;
    %Link Motor Inertia
    Jm = zeros(7,1);
    Jm(1) = 0.00011631;
    Jm(2) = 0.00011831;
    Jm(3) = 0.00011831;
    Jm(4) = 0.00010686;
    Jm(5) = 0.00001685;
    Jm(6) = 0.00001745;
    Jm(7) = 0.00000142;
             
    if hand_on
        hand_mass = 1.3731;
        DH_d(7) = DH_d(7) + .0953; % Adding the distance to the hand frame for the Schunk Gripper
        com(:,7) = ([0.001127;	-0.000211;	0.054851].*hand_mass + com(:,7).*m(7))/(hand_mass + m(7)); % Finding the combined center of mass
        m(7) = m(7) + hand_mass; % Adding the mass of the hand
        I(:,:,7) = [ .003167342,          0,         0;       % Approximate Inertia Tensor for Schunk Gripper
                              0, .001128942,         0;
                              0,          0, .00258007;];
    end
    
%-------------------------------------------------------------------------------------
%  END SETUP OF THE ARM
%-------------------------------------------------------------------------------------

    z0 = [0;0;1];
    grav = [0 0 9.81];
	fext = zeros(6, 1);
    n = 7;
    FTsensor = zeros(6,1);
    
    tau = zeros(n,1);
    
    Fm = zeros(3,7);
    Nm = zeros(3,7);
    N = zeros(3,1);
    pstarm = zeros(3,7);
    Rm = zeros(3,3,7);
    w = zeros(3,1);
    wd = zeros(3,1);
    v = zeros(3,1);
    vd = grav(:);
    
    
    %
	% init some variables, compute the link rotation matrices
	%
    for j=1:n,
        a = DH_a(j);
        d = DH_d(j);
        alpha = DH_alpha(j);
        Tj = getTransformDH(a, d, alpha, q(j));
        
        pstar = [a; d*sin(alpha); d*cos(alpha)];
        if j == 1,
            pstar = eye(3) * pstar;
            Tj = eye(4) * Tj;
        end
        pstarm(:,j) = pstar;
        Rm(:,:,j) = Tj(1:3,1:3);
    end
    
    %
	%  the forward recursion
	%
    for j=1:n,
        Rt = Rm(:,:,j)';	% transpose!!
        pstar = pstarm(:,j);
        r = com(:,j)';

        %
        % statement order is important here
        %
        % revolute axis
        wd = Rt*(wd + z0*qdd(j) + cross(w,z0*qd(j)));
        w = Rt*(w + z0*qd(j));
        %v = cross(w,pstar) + Rt*v;
        vd = cross(wd,pstar) + cross(w, cross(w,pstar)) + Rt*vd;

        %vhat = cross(wd,r') + cross(w,cross(w,r')) + vd;
        vhat = cross(wd,r') + cross(w,cross(w,r')) + vd;
        F = m(j)*vhat;
        N = I(1:3,1:3,j)*wd + cross(w,I(1:3,1:3,j)*w);
        Fm(:,j) = F;
        Nm(:,j) = N;
    end
    
    
    %
	%  the backward recursion
	%

    fext = fext(:);
    f = fext(1:3);		% force/moments on end of arm
    nn = fext(4:6);

    for j=n:-1:1,
        pstar = pstarm(:,j);

        %
        % order of these statements is important, since both
        % nn and f are functions of previous f.
        %
        if j == n,
            R = eye(3,3);
        else
            R = Rm(:,:,j+1);
        end
        r = com(:,j)';
        
        % The expected force/torque at the sensor.  Used for dynamic compensation
        % of the gripper.
        if j == n
            FTsensor(1:3) = R*f + Fm(:,j);
            FTsensor(4:6) = cross(r',Fm(:,j));
        end
        
        nn = R*(nn + cross(R'*pstar,f)) + cross(pstar+r',Fm(:,j)) + Nm(:,j);
        f = R*f + Fm(:,j);
        
        R = Rm(:,:,j);
        % revolute
        tau(j) = nn'*(R'*z0) + G(j)^2 * Jm(j)*qdd(j);% + abs(G(j)) * friction(link, qd(j));
    end

end

function T = getTransformDH(a,d,alpha,q)
    ct = cos(q);
    st = sin(q);
    cb = cos(alpha);
    sb = sin(alpha);
    
    T = [ ct, -st*cb,  st*sb, a*ct;
          st,  ct*cb, -ct*sb, a*st;
          0, sb, cb, d;
          0, 0, 0, 1 ];
end
